simulink model "impedancia"  (R2017b)
settings: Solver=VariableStepAuto  StartTime=0.0  StopTime=3  RelTol=1e-3
libraries: roblocks x6, simulink x1
settings Model: Creator=USUARIO  LastModifiedBy=USUARIO

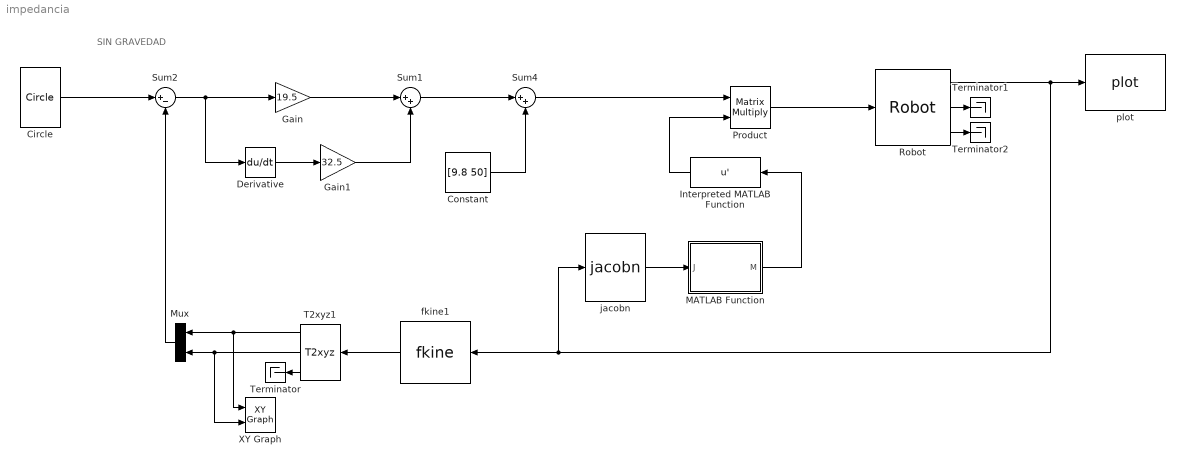
== system impedancia ==
  note: SIN GRAVEDAD
  Circle : roblocks/Toolbox/Circle  radius=1  freq=4
  Constant : Constant  Value=[9.8 50]  VectorParams1D=off
  Derivative : Derivative
  Gain : Gain  Gain=19.5
  Gain1 : Gain  Gain=32.5
  Interpreted MATLAB Function : MATLABFcn  MATLABFcn=u'  OutputDimensions=[2 2]  Output1D=off
  MATLAB Function : MATLAB Function  TreatAsAtomicUnit=on
  Mux : Mux  Inputs=2
  Product : Product  Multiplication=Matrix(*)
  Robot : roblocks/Arm/Robot  robot=Robot  q0=[pi/2 pi/2]
  Sum1 : Sum  Inputs=|++
  Sum2 : Sum  Inputs=|+-
  Sum4 : Sum  Inputs=|++
  T2xyz1 : roblocks/Toolbox/T2xyz
  Terminator : Terminator
  Terminator1 : Terminator
  Terminator2 : Terminator
  XY Graph : simulink/Sinks/XY Graph  xmin=-30  xmax=50  ymin=-50  ymax=30  st=-1
  fkine1 : roblocks/Arm/fkine  robot=Robot
  jacobn : roblocks/Arm/jacobn  robot=Robot
  plot : roblocks/Arm/plot  robot=Robot  fps=5  holdplot=on
  wires:
  Sum2/1 -> Derivative/1, Gain/1
  Derivative/1 -> Gain1/1
  Gain/1 -> Sum1/1
  Gain1/1 -> Sum1/2
  Sum1/1 -> Sum4/1
  Robot/1 -> plot/1, jacobn/1, fkine1/1
  Product/1 -> Robot/1
  T2xyz1/1 -> XY Graph/1, Mux/1
  T2xyz1/2 -> XY Graph/2, Mux/2
  Mux/1 -> Sum2/2
  Constant/1 -> Sum4/2
  T2xyz1/3 -> Terminator/1
  Robot/2 -> Terminator1/1
  Robot/3 -> Terminator2/1
  fkine1/1 -> T2xyz1/1
  Sum4/1 -> Product/1
  Circle/1 -> Sum2/1
  MATLAB Function/1(M) -> Interpreted MATLAB Function/1
  Interpreted MATLAB Function/1 -> Product/2
  jacobn/1 -> MATLAB Function/1(J)

== matlab function impedancia/MATLAB Function ==
  data: J input; M output
function M = fcn(J)
M=J(2:3,1:2);
